simulink model "old_triad"  (R2025a)
settings: Solver=VariableStepAuto  StartTime=0.0  StopTime=10.0  RelTol=1e-3
libraries: vrlib x8
settings Model: Creator=procyon  LastModifiedBy=procyon

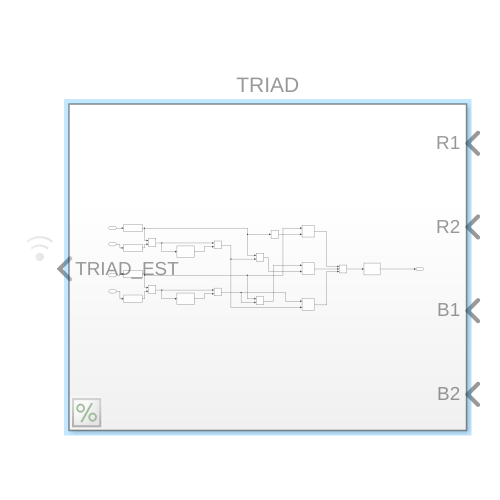
[thumbnail: Simulink's stored preview of the top-level diagram]
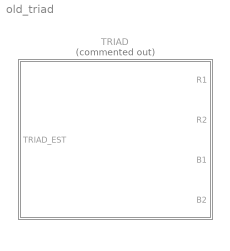
== system old_triad ==
  TRIAD : Subsystem  Commented=on

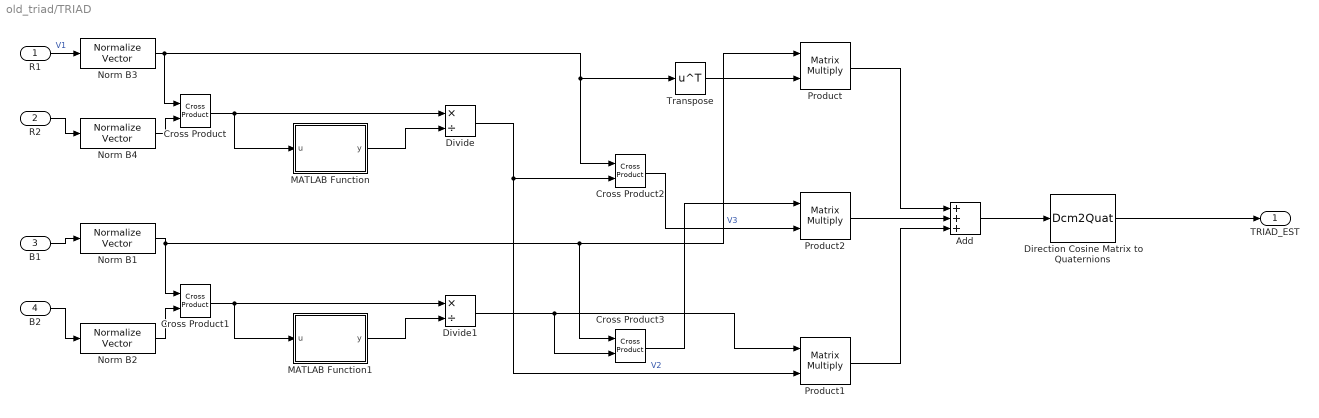
== system old_triad/TRIAD ==
  R1 : Inport
  R2 : Inport  Port=2
  B1 : Inport  Port=3
  B2 : Inport  Port=4
  Add : Sum  Inputs=+++
  Cross Product{,1..3} (4 alike) : vrlib/Utilities/Cross Product
  Direction Cosine Matrix to Quaternions : Dcm2Quat  action=Warning
  Divide : Product  Inputs=*/
  Divide1 : Product  Inputs=*/
  MATLAB Function : MATLAB Function  TreatAsAtomicUnit=on
  MATLAB Function1 : MATLAB Function  TreatAsAtomicUnit=on
  Norm B{1..4} (4 alike) : vrlib/Utilities/Normalize Vector  maxzero=0
  Product : Product  Multiplication=Matrix(*)
  Product1 : Product  Multiplication=Matrix(*)
  Product2 : Product  Multiplication=Matrix(*)
  Transpose : Math  Operator=transpose
  TRIAD_EST : Outport
  wires:
  Direction Cosine Matrix to Quaternions/1 -> TRIAD_EST/1
  R1/1 -> Norm B3/1  "V1"
  Cross Product/1 -> MATLAB Function/1(u), Divide/1
  MATLAB Function/1(y) -> Divide/2
  Cross Product1/1 -> MATLAB Function1/1(u), Divide1/1
  B1/1 -> Norm B1/1
  MATLAB Function1/1(y) -> Divide1/2
  B2/1 -> Norm B2/1
  Divide/1 -> Product1/2, Cross Product2/2  "V2"
  Divide1/1 -> Product1/1, Cross Product3/2
  Transpose/1 -> Product/2
  Cross Product3/1 -> Product2/1
  Cross Product2/1 -> Product2/2  "V3"
  Product2/1 -> Add/2
  Product/1 -> Add/1
  Product1/1 -> Add/3
  Add/1 -> Direction Cosine Matrix to Quaternions/1
  R2/1 -> Norm B4/1
  Norm B2/1 -> Cross Product1/2
  Norm B1/1 -> Product/1, Cross Product3/1, Cross Product1/1
  Norm B3/1 -> Transpose/1, Cross Product2/1, Cross Product/1
  Norm B4/1 -> Cross Product/2

== matlab function old_triad/TRIAD/MATLAB Function1 ==
  data: u input; y output
function y = l2norm(u)
%#codegen
% Euclidean (L2) norm of a vector u
% Works for row or column vectors (double/single)

u = u(:);                  % force column
y = sqrt(sum(u .* u));     % ||u||_2 = sqrt(u'u)
end

== matlab function old_triad/TRIAD/MATLAB Function ==
  data: u input; y output
function y = l2norm(u)
%#codegen
% Euclidean (L2) norm of a vector u
% Works for row or column vectors (double/single)

u = u(:);                  % force column
y = sqrt(sum(u .* u));     % ||u||_2 = sqrt(u'u)
end
